simulink model "cordicSynth0"  (R2020b)
settings: Solver=FixedStepDiscrete  StartTime=0.0  StopTime=10.0  RelTol=1e-3
values from neighbouring files (symbols this model uses):
  cordicIter = cordicIterParam(m)    [readAreaReport.m]    (also in run_cordic_hdlworkflow.m)
libraries: simulink x1
settings Model: DataTypeOverride=Off  Creator=amatsumo  LastModifiedBy=amatsumo
settings DataIOCC: SaveOutput=off  SaveTime=off
settings OptimizationCC: BlockReduction=off  ConditionallyExecuteInputs=off  DefaultParameterBehavior=Inlined
settings DebuggingCC: AlgebraicLoopMsg=error  SingleTaskRateTransMsg=error  StrictBusMsg=ErrorOnBusTreatedAsVector  ArithmeticOperatorsInVariantConditions=warning
settings HardwareCC: ProdBitPerPointer=32  ProdBitPerSizeT=32  ProdBitPerPtrDiffT=32  ProdLargestAtomicFloat=None  ProdIntDivRoundTo=Undefined  ProdEndianess=Unspecified  ProdWordSize=32  ProdHWDeviceType=ASIC/FPGA->ASIC/FPGA  ProdEqTarget=off
settings SFSimCC: SimUseLocalCustomCode=off  CustomCodeUndefinedFunction=UseInterfaceOnly
settings RTWCC: RTWUseLocalCustomCode=off
settings CodeAppCC: StateflowObjectComments=on
settings GRTTargetCC: TargetLangStandard=C89/C90 (ANSI)

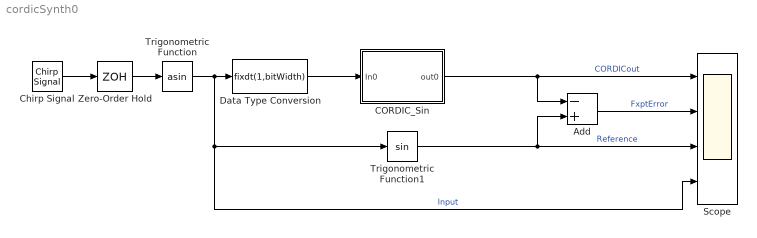
== system cordicSynth0 ==
  Add : Sum  Inputs=-+  AccumDataTypeStr=double  OutDataTypeStr=double
  CORDIC_Sin : Subsystem
  Chirp Signal : simulink/Sources/Chirp Signal  f1=1  T=10  f2=100
  Data Type Conversion : DataTypeConversion  OutMin=-1.566  OutMax=1.566  OutDataTypeStr=fixdt(1,bitWidth)  RndMeth=Nearest
  Scope : Scope  NumInputPorts=4
  Trigonometric Function : Trigonometry  Operator=asin
  Trigonometric Function1 : Trigonometry  NumberOfIterations=8
  Zero-Order Hold : ZeroOrderHold  SampleTime=1/1000
  wires:
  Chirp Signal/1 -> Zero-Order Hold/1
  Zero-Order Hold/1 -> Trigonometric Function/1
  Trigonometric Function1/1 -> Add/2, Scope/3  "Reference"
  Trigonometric Function/1 -> Trigonometric Function1/1, Scope/4, Data Type Conversion/1  "Input"
  CORDIC_Sin/1(out0) -> Add/1, Scope/1  "CORDICout"
  Data Type Conversion/1 -> CORDIC_Sin/1(In0)
  Add/1 -> Scope/2  "FxptError"

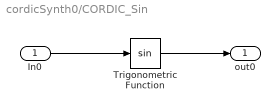
== system cordicSynth0/CORDIC_Sin ==
  In0 : Inport
  Trigonometric Function : Trigonometry  ApproximationMethod=CORDIC  NumberOfIterations=cordicIter
  out0 : Outport
  wires:
  In0/1 -> Trigonometric Function/1
  Trigonometric Function/1 -> out0/1
